simulink model "sys_model"  (R2015a)
settings: configuration reference "config_cosim" (kept outside this file)
InitFcn:
  | h  = findall(0, 'tag','Display');
  | close(h)
  | load TestVel
StartFcn:
  | Display
StopFcn:
  | h  = findall(0, 'tag','Display');
  | %close(h)
undefined symbols (not defined in the file): Vmsl, Vtgt
(part 1 of 2)
settings Model: CovModelRefEnable=off  Creator=The MathWorks, Inc.  LastModifiedBy=ericli
settings ConfigSetRef: SourceLocation=Base Workspace

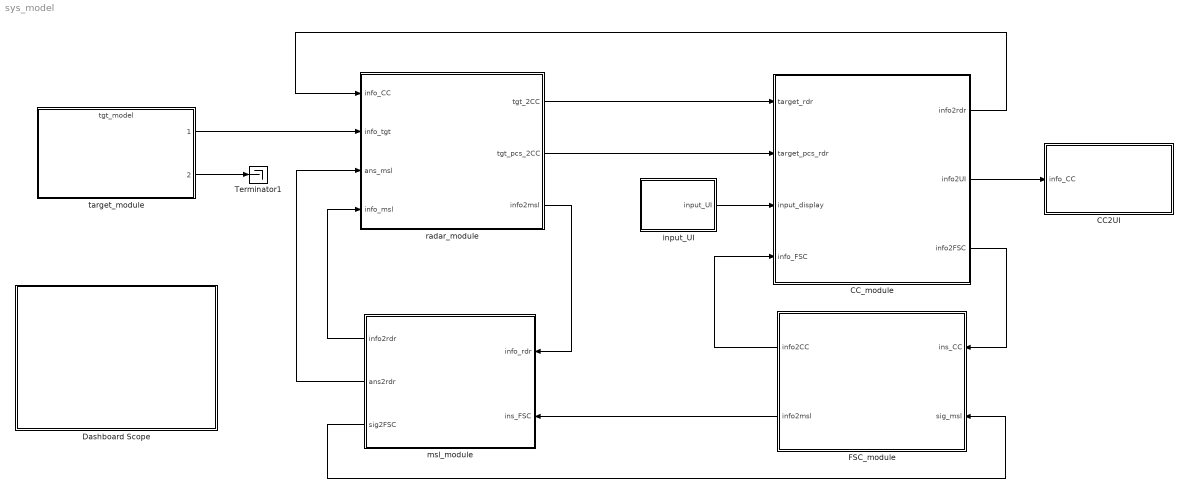
== system sys_model ==
  CC2UI : Subsystem
  CC_module : Subsystem
  Dashboard Scope : Subsystem  DialogController=hmiCreateDDGDialog  IsWebBlock=on  mask(MathWorksWebBlock){webBlockId=861919ea-88f4-4d9a-9fd6-bc31e51d36de, webBlockType=sdiscope, ShowInitialText=on, HMISrcModelName=sys_model}
      mask prompts: webBlockId "WebBlock Id"; webBlockType "WebBlock Type"; HMISrcModelName "Source Model"
      mask Help: helpview([docroot '/mapfiles/simulink.map'], 'hmi_scope')
      mask Display:
      | if strcmp(get_param(bdroot(gcb),'BlockDiagramType'), 'library')
      |     image([(matlabroot) '/toolbox/simulink/hmi/icons/DashboardScope.png']);
      | end
  FSC_module : Subsystem
  Terminator1 : Terminator
  input_UI : Subsystem
  msl_module : Subsystem
  radar_module : Subsystem
  target_module : ModelReference  ModelNameDialog=tgt_model.slx  SimulationMode=Normal  ModelReferenceVersion=1.185  CopyOfModelName=tgt_model.slx  DefaultDataLogging=on
  wires:
  target_module/1 -> radar_module/2(info_tgt)
  FSC_module/2(info2msl) -> msl_module/2(ins_FSC)
  CC_module/2(info2UI) -> CC2UI/1(info_CC)
  radar_module/3(info2msl) -> msl_module/1(info_rdr)
  msl_module/1(info2rdr) -> radar_module/4(info_msl)
  FSC_module/1(info2CC) -> CC_module/4(info_FSC)
  CC_module/1(info2rdr) -> radar_module/1(info_CC)
  target_module/2 -> Terminator1/1
  input_UI/1(input_UI) -> CC_module/3(input_display)
  msl_module/2(ans2rdr) -> radar_module/3(ans_msl)
  msl_module/3(sig2FSC) -> FSC_module/2(sig_msl)
  CC_module/3(info2FSC) -> FSC_module/1(ins_CC)
  radar_module/1(tgt_2CC) -> CC_module/1(target_rdr)
  radar_module/2(tgt_pcs_2CC) -> CC_module/2(target_pcs_rdr)

== system sys_model/CC2UI ==
  info_CC : Inport
  Bus Selector : BusSelector  OutputSignals=TargetData,AsnData,StateData,Avl_info,MslMotion
  Model : ModelReference  ModelNameDialog=SetData.slx  SimulationMode=Normal  ModelReferenceVersion=1.204  CopyOfModelName=SetData.slx  DefaultDataLogging=on
  wires:
  info_CC/1 -> Bus Selector/1
  Bus Selector/1 -> Model/1  "<TargetData>"
  Bus Selector/2 -> Model/2  "<AsnData>"
  Bus Selector/3 -> Model/3  "<StateData>"
  Bus Selector/4 -> Model/4  "<Avl_info>"
  Bus Selector/5 -> Model/5  "<MslMotion>"

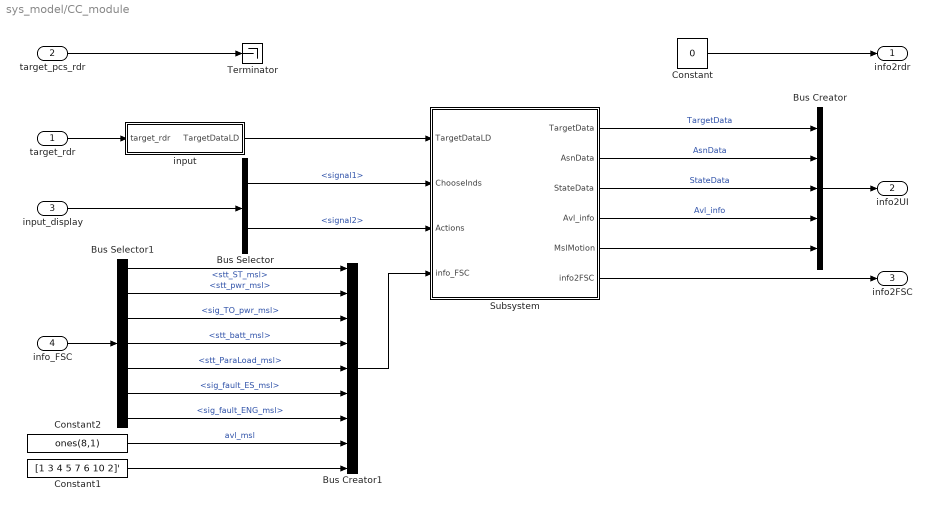
== system sys_model/CC_module ==
  target_rdr : Inport  OutDataTypeStr=Bus: BusObject_tgt_rdr2CC
  target_pcs_rdr : Inport  Port=2
  input_display : Inport  Port=3
  info_FSC : Inport  Port=4  OutDataTypeStr=Bus: BusObject_info_FSC2CC
  Bus Creator : BusCreator  Inputs=5
  Bus Creator1 : BusCreator  Inputs=9  OutDataTypeStr=Bus: BusObject_info_FSC2CC
  Bus Selector : BusSelector  OutputSignals=signal1,signal2
  Bus Selector1 : BusSelector  OutputSignals=stt_ST_msl,stt_pwr_msl,sig_TO_pwr_msl,stt_batt_msl,stt_ParaLoad_msl,sig_fault_ES_msl,sig_fault_ENG_msl
  Constant : Constant  Value=0  OutDataTypeStr=Bus:BusObject_info_CC2rdr  LockScale=on
  Constant1 : Constant  Value=[1 3 4 5 7 6 10 2]'  OutDataTypeStr=double
  Constant2 : Constant  Value=ones(8,1)  OutDataTypeStr=boolean
  Subsystem : Subsystem
  Terminator : Terminator
  input : Subsystem
  info2rdr : Outport  OutDataTypeStr=Bus: BusObject_info_CC2rdr
  info2UI : Outport  Port=2
  info2FSC : Outport  Port=3  OutDataTypeStr=Bus: BusObject_info_CC2FSC
  wires:
  Bus Creator/1 -> info2UI/1
  input_display/1 -> Bus Selector/1
  Bus Selector/2 -> Subsystem/3(Actions)  "<signal2>"
  Subsystem/6(info2FSC) -> info2FSC/1
  Constant/1 -> info2rdr/1
  Subsystem/4(Avl_info) -> Bus Creator/4  "Avl_info"
  Subsystem/3(StateData) -> Bus Creator/3  "StateData"
  Subsystem/1(TargetData) -> Bus Creator/1  "TargetData"
  input/1(TargetDataLD) -> Subsystem/1(TargetDataLD)
  target_pcs_rdr/1 -> Terminator/1
  Subsystem/2(AsnData) -> Bus Creator/2  "AsnData"
  info_FSC/1 -> Bus Selector1/1
  Bus Selector1/1 -> Bus Creator1/1  "<stt_ST_msl>"
  Bus Selector1/3 -> Bus Creator1/3  "<sig_TO_pwr_msl>"
  Bus Selector1/4 -> Bus Creator1/4  "<stt_batt_msl>"
  Bus Selector1/5 -> Bus Creator1/5  "<stt_ParaLoad_msl>"
  Bus Selector1/6 -> Bus Creator1/6  "<sig_fault_ES_msl>"
  Bus Selector1/7 -> Bus Creator1/7  "<sig_fault_ENG_msl>"
  Constant2/1 -> Bus Creator1/8  "avl_msl"
  Constant1/1 -> Bus Creator1/9
  Bus Creator1/1 -> Subsystem/4(info_FSC)
  target_rdr/1 -> input/1(target_rdr)
  Bus Selector/1 -> Subsystem/2(ChooseInds)  "<signal1>"
  Subsystem/5(MslMotion) -> Bus Creator/5
  Bus Selector1/2 -> Bus Creator1/2  "<stt_pwr_msl>"

== system sys_model/Dashboard Scope ==

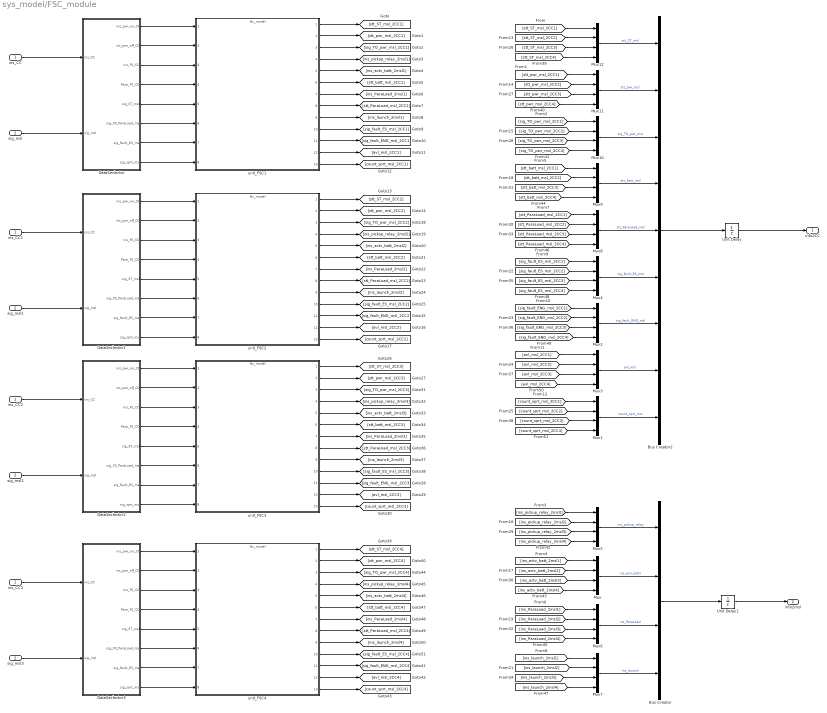
== system sys_model/FSC_module ==
  ins_CC : Inport
  sig_msl : Inport  Port=2
  Bus Creator : BusCreator  OutDataTypeStr=Bus: BusObject_info_FSC2msl  NonVirtualBus=on
      settings: InheritFromInputs=off
  Bus Creator2 : BusCreator  Inputs=9  OutDataTypeStr=Bus: BusObject_info_FSC2CC  NonVirtualBus=on
      settings: InheritFromInputs=off
  DataSeclector : Subsystem
  DataSeclector1 : Subsystem
  DataSeclector2 : Subsystem
  DataSeclector3 : Subsystem
  Mux{,1..12} (13 alike) : Mux
  Unit Delay : UnitDelay  SampleTime=-1
  Unit Delay1 : UnitDelay  SampleTime=-1
  ins_CC1 : InportShadow
  ins_CC2 : InportShadow
  ins_CC3 : InportShadow
  sig_msl1 : InportShadow  Port=2
  sig_msl2 : InportShadow  Port=2
  sig_msl3 : InportShadow  Port=2
  unit_FSC{1..4} (4 alike) : ModelReference  ModelNameDialog=fsc_model.slx  SimulationMode=Normal  ModelReferenceVersion=1.143  CopyOfModelName=fsc_model.slx  DefaultDataLogging=on
  info2CC : Outport  OutDataTypeStr=Bus: BusObject_info_FSC2CC
  info2msl : Outport  Port=2  OutDataTypeStr=Bus: BusObject_info_FSC2msl
  wires:
  unit_FSC1/1 -> [stt_ST_msl_2CC1]
  unit_FSC1/2 -> [stt_pwr_msl_2CC1]
  unit_FSC1/3 -> [sig_TO_pwr_msl_2CC1]
  unit_FSC1/4 -> [ins_pickup_relay_2msl1]
  unit_FSC1/5 -> [ins_actv_batt_2msl1]
  unit_FSC1/6 -> [stt_batt_msl_2CC1]
  unit_FSC1/7 -> [ins_ParaLoad_2msl1]
  unit_FSC1/8 -> [stt_ParaLoad_msl_2CC1]
  unit_FSC1/9 -> [ins_launch_2msl1]
  unit_FSC1/10 -> [sig_fault_ES_msl_2CC1]
  unit_FSC1/11 -> [sig_fault_ENG_msl_2CC1]
  unit_FSC1/12 -> [avl_msl_2CC1]
  unit_FSC1/13 -> [count_sprt_msl_2CC1]
  unit_FSC2/13 -> [count_sprt_msl_2CC2]
  unit_FSC2/6 -> [stt_batt_msl_2CC2]
  unit_FSC2/10 -> [sig_fault_ES_msl_2CC2]
  unit_FSC2/3 -> [sig_TO_pwr_msl_2CC2]
  unit_FSC2/7 -> [ins_ParaLoad_2msl2]
  unit_FSC2/11 -> [sig_fault_ENG_msl_2CC2]
  unit_FSC2/4 -> [ins_pickup_relay_2msl2]
  unit_FSC2/8 -> [stt_ParaLoad_msl_2CC2]
  unit_FSC2/1 -> [stt_ST_msl_2CC2]
  unit_FSC2/2 -> [stt_pwr_msl_2CC2]
  unit_FSC2/9 -> [ins_launch_2msl2]
  unit_FSC2/12 -> [avl_msl_2CC2]
  unit_FSC2/5 -> [ins_actv_batt_2msl2]
  unit_FSC3/11 -> [sig_fault_ENG_msl_2CC3]
  unit_FSC3/7 -> [ins_ParaLoad_2msl3]
  unit_FSC3/4 -> [ins_pickup_relay_2msl3]
  unit_FSC3/10 -> [sig_fault_ES_msl_2CC3]
  unit_FSC3/5 -> [ins_actv_batt_2msl3]
  unit_FSC3/6 -> [stt_batt_msl_2CC3]
  unit_FSC3/3 -> [sig_TO_pwr_msl_2CC3]
  unit_FSC3/1 -> [stt_ST_msl_2CC3]
  unit_FSC3/13 -> [count_sprt_msl_2CC3]
  unit_FSC3/12 -> [avl_msl_2CC3]
  unit_FSC3/2 -> [stt_pwr_msl_2CC3]
  unit_FSC3/9 -> [ins_launch_2msl3]
  unit_FSC3/8 -> [stt_ParaLoad_msl_2CC3]
  unit_FSC4/11 -> [sig_fault_ENG_msl_2CC4]
  unit_FSC4/12 -> [avl_msl_2CC4]
  unit_FSC4/10 -> [sig_fault_ES_msl_2CC4]
  unit_FSC4/9 -> [ins_launch_2msl4]
  unit_FSC4/8 -> [stt_ParaLoad_msl_2CC4]
  unit_FSC4/7 -> [ins_ParaLoad_2msl4]
  unit_FSC4/6 -> [stt_batt_msl_2CC4]
  unit_FSC4/5 -> [ins_actv_batt_2msl4]
  unit_FSC4/4 -> [ins_pickup_relay_2msl4]
  unit_FSC4/3 -> [sig_TO_pwr_msl_2CC4]
  unit_FSC4/1 -> [stt_ST_msl_2CC4]
  unit_FSC4/2 -> [stt_pwr_msl_2CC4]
  unit_FSC4/13 -> [count_sprt_msl_2CC4]
  [stt_ST_msl_2CC1] -> Mux12/1
  [stt_ST_msl_2CC2] -> Mux12/2
  [stt_ST_msl_2CC3] -> Mux12/3
  [stt_ST_msl_2CC4] -> Mux12/4
  [stt_pwr_msl_2CC1] -> Mux11/1
  [stt_pwr_msl_2CC2] -> Mux11/2
  [stt_pwr_msl_2CC3] -> Mux11/3
  [stt_pwr_msl_2CC4] -> Mux11/4
  [sig_TO_pwr_msl_2CC1] -> Mux10/1
  [sig_TO_pwr_msl_2CC2] -> Mux10/2
  [sig_TO_pwr_msl_2CC3] -> Mux10/3
  [sig_TO_pwr_msl_2CC4] -> Mux10/4
  [ins_pickup_relay_2msl1] -> Mux5/1
  [ins_pickup_relay_2msl2] -> Mux5/2
  [ins_pickup_relay_2msl3] -> Mux5/3
  [ins_pickup_relay_2msl4] -> Mux5/4
  [ins_actv_batt_2msl1] -> Mux/1
  [ins_actv_batt_2msl2] -> Mux/2
  [ins_actv_batt_2msl3] -> Mux/3
  [ins_actv_batt_2msl4] -> Mux/4
  [stt_batt_msl_2CC1] -> Mux9/1
  [stt_batt_msl_2CC2] -> Mux9/2
  [stt_batt_msl_2CC3] -> Mux9/3
  [stt_batt_msl_2CC4] -> Mux9/4
  [ins_ParaLoad_2msl1] -> Mux6/1
  [ins_ParaLoad_2msl2] -> Mux6/2
  [ins_ParaLoad_2msl3] -> Mux6/3
  [ins_ParaLoad_2msl4] -> Mux6/4
  [stt_ParaLoad_msl_2CC1] -> Mux8/1
  [stt_ParaLoad_msl_2CC2] -> Mux8/2
  [stt_ParaLoad_msl_2CC3] -> Mux8/3
  [stt_ParaLoad_msl_2CC4] -> Mux8/4
  [ins_launch_2msl1] -> Mux7/1
  [ins_launch_2msl2] -> Mux7/2
  [ins_launch_2msl3] -> Mux7/3
  [ins_launch_2msl4] -> Mux7/4
  [sig_fault_ES_msl_2CC1] -> Mux4/1
  [sig_fault_ES_msl_2CC2] -> Mux4/2
  [sig_fault_ES_msl_2CC3] -> Mux4/3
  [sig_fault_ES_msl_2CC4] -> Mux4/4
  [sig_fault_ENG_msl_2CC1] -> Mux2/1
  [sig_fault_ENG_msl_2CC2] -> Mux2/2
  [sig_fault_ENG_msl_2CC3] -> Mux2/3
  [sig_fault_ENG_msl_2CC4] -> Mux2/4
  [avl_msl_2CC1] -> Mux3/1
  [avl_msl_2CC2] -> Mux3/2
  [avl_msl_2CC3] -> Mux3/3
  [avl_msl_2CC4] -> Mux3/4
  [count_sprt_msl_2CC1] -> Mux1/1
  [count_sprt_msl_2CC2] -> Mux1/2
  [count_sprt_msl_2CC3] -> Mux1/3
  [count_sprt_msl_2CC4] -> Mux1/4
  Mux6/1 -> Bus Creator/3  "ins_ParaLoad"
  Mux/1 -> Bus Creator/2  "ins_actv_batt"
  Mux7/1 -> Bus Creator/4  "ins_launch"
  Mux5/1 -> Bus Creator/1  "ins_pickup_relay"
  Bus Creator/1 -> Unit Delay1/1
  Mux10/1 -> Bus Creator2/3  "sig_TO_pwr_msl"
  Mux9/1 -> Bus Creator2/4  "stt_batt_msl"
  Mux11/1 -> Bus Creator2/2  "stt_pwr_msl"
  Mux8/1 -> Bus Creator2/5  "stt_ParaLoad_msl"
  Mux4/1 -> Bus Creator2/6  "sig_fault_ES_msl"
  Mux12/1 -> Bus Creator2/1  "stt_ST_msl"
  Mux2/1 -> Bus Creator2/7  "sig_fault_ENG_msl"
  Mux3/1 -> Bus Creator2/8  "avl_msl"
  Mux1/1 -> Bus Creator2/9  "count_sprt_msl"
  Bus Creator2/1 -> Unit Delay/1
  ins_CC/1 -> DataSeclector/1(ins_CC)
  sig_msl/1 -> DataSeclector/2(sig_msl)
  DataSeclector/3(ins_FS_CC) -> unit_FSC1/3
  DataSeclector/2(ins_pwr_off_CC) -> unit_FSC1/2
  DataSeclector/4(Para_FS_CC) -> unit_FSC1/4
  DataSeclector/5(sig_ST_msl) -> unit_FSC1/5
  DataSeclector/1(ins_pwr_on_CC) -> unit_FSC1/1
  DataSeclector/6(sig_CK_ParaLoad_msl) -> unit_FSC1/6
  DataSeclector/7(sig_fault_ES_msl) -> unit_FSC1/7
  DataSeclector/8(sig_sprt_msl) -> unit_FSC1/8
  DataSeclector3/6(sig_CK_ParaLoad_msl) -> unit_FSC4/6
  DataSeclector3/2(ins_pwr_off_CC) -> unit_FSC4/2
  DataSeclector3/5(sig_ST_msl) -> unit_FSC4/5
  DataSeclector3/8(sig_sprt_msl) -> unit_FSC4/8
  DataSeclector3/4(Para_FS_CC) -> unit_FSC4/4
  DataSeclector3/3(ins_FS_CC) -> unit_FSC4/3
  DataSeclector3/1(ins_pwr_on_CC) -> unit_FSC4/1
  DataSeclector3/7(sig_fault_ES_msl) -> unit_FSC4/7
  DataSeclector2/4(Para_FS_CC) -> unit_FSC3/4
  DataSeclector2/2(ins_pwr_off_CC) -> unit_FSC3/2
  DataSeclector2/1(ins_pwr_on_CC) -> unit_FSC3/1
  DataSeclector2/5(sig_ST_msl) -> unit_FSC3/5
  DataSeclector2/3(ins_FS_CC) -> unit_FSC3/3
  DataSeclector2/7(sig_fault_ES_msl) -> unit_FSC3/7
  DataSeclector2/8(sig_sprt_msl) -> unit_FSC3/8
  DataSeclector2/6(sig_CK_ParaLoad_msl) -> unit_FSC3/6
  DataSeclector1/8(sig_sprt_msl) -> unit_FSC2/8
  DataSeclector1/1(ins_pwr_on_CC) -> unit_FSC2/1
  DataSeclector1/6(sig_CK_ParaLoad_msl) -> unit_FSC2/6
  DataSeclector1/4(Para_FS_CC) -> unit_FSC2/4
  DataSeclector1/3(ins_FS_CC) -> unit_FSC2/3
  DataSeclector1/5(sig_ST_msl) -> unit_FSC2/5
  DataSeclector1/7(sig_fault_ES_msl) -> unit_FSC2/7
  DataSeclector1/2(ins_pwr_off_CC) -> unit_FSC2/2
  sig_msl1/1 -> DataSeclector1/2(sig_msl)
  ins_CC1/1 -> DataSeclector1/1(ins_CC)
  ins_CC2/1 -> DataSeclector2/1(ins_CC)
  sig_msl2/1 -> DataSeclector2/2(sig_msl)
  sig_msl3/1 -> DataSeclector3/2(sig_msl)
  ins_CC3/1 -> DataSeclector3/1(ins_CC)
  Unit Delay/1 -> info2CC/1
  Unit Delay1/1 -> info2msl/1

== system sys_model/input_UI ==
  " get_input_UI" : ModelReference  ModelNameDialog=input_display.slx  SimulationMode=Normal  ModelReferenceVersion=1.222  CopyOfModelName=input_display.slx  DefaultDataLogging=on
  Bus Creator : BusCreator  Inputs=2
  input_UI : Outport
  wires:
  Bus Creator/1 -> input_UI/1
  " get_input_UI"/1 -> Bus Creator/1
  " get_input_UI"/2 -> Bus Creator/2

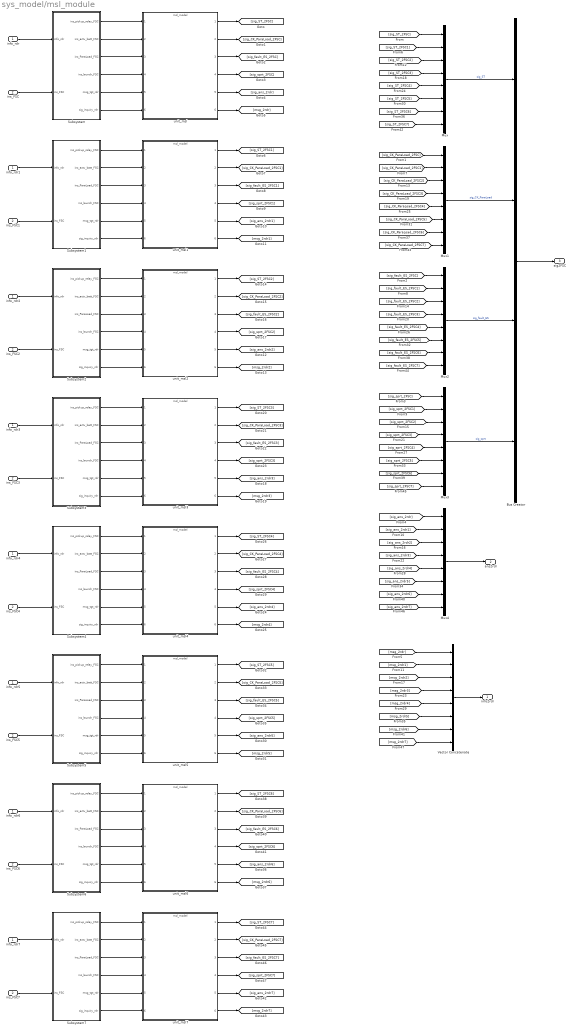
== system sys_model/msl_module ==
  info_rdr : Inport
  ins_FSC : Inport  Port=2
  Bus Creator : BusCreator
  Mux{,1..4} (5 alike) : Mux  Inputs=8
  Subsystem : Subsystem
  Subsystem1 : Subsystem
  Subsystem2 : Subsystem
  Subsystem3 : Subsystem
  Subsystem4 : Subsystem
  Subsystem5 : Subsystem
  Subsystem6 : Subsystem
  Subsystem7 : Subsystem
  Vector Concatenate : Concatenate  NumInputs=8
  info_rdr{1..7} (7 alike) : InportShadow
  ins_FSC{1..7} (7 alike) : InportShadow  Port=2
  unit_msl{,1..7} (8 alike) : ModelReference  ModelNameDialog=msl_model.slx  SimulationMode=Normal  ModelReferenceVersion=1.166  CopyOfModelName=msl_model.slx  DefaultDataLogging=on
  info2rdr : Outport  OutDataTypeStr=Bus: BusObject_msg_msl2rdr
  ans2rdr : Outport  Port=2
  sig2FSC : Outport  Port=3  OutDataTypeStr=Bus: BusObject_info_msl2FSC
  wires:
  ins_FSC/1 -> Subsystem/2(ins_FSC)
  info_rdr/1 -> Subsystem/1(info_rdr)
  Subsystem/1(ins_pickup_relay_FSC) -> unit_msl/1
  Subsystem/2(ins_actv_batt_FSC) -> unit_msl/2
  Subsystem/3(ins_ParaLoad_FSC) -> unit_msl/3
  Subsystem/4(ins_launch_FSC) -> unit_msl/4
  Subsystem/5(msg_tgt_rdr) -> unit_msl/5
  Subsystem/6(sig_inquiry_rdr) -> unit_msl/6
  ins_FSC1/1 -> Subsystem1/2(ins_FSC)
  info_rdr1/1 -> Subsystem1/1(info_rdr)
  Subsystem1/1(ins_pickup_relay_FSC) -> unit_msl1/1
  Subsystem1/2(ins_actv_batt_FSC) -> unit_msl1/2
  Subsystem1/3(ins_ParaLoad_FSC) -> unit_msl1/3
  Subsystem1/4(ins_launch_FSC) -> unit_msl1/4
  Subsystem1/5(msg_tgt_rdr) -> unit_msl1/5
  Subsystem1/6(sig_inquiry_rdr) -> unit_msl1/6
  ins_FSC2/1 -> Subsystem2/2(ins_FSC)
  info_rdr2/1 -> Subsystem2/1(info_rdr)
  Subsystem2/1(ins_pickup_relay_FSC) -> unit_msl2/1
  Subsystem2/2(ins_actv_batt_FSC) -> unit_msl2/2
  Subsystem2/3(ins_ParaLoad_FSC) -> unit_msl2/3
  Subsystem2/4(ins_launch_FSC) -> unit_msl2/4
  Subsystem2/5(msg_tgt_rdr) -> unit_msl2/5
  Subsystem2/6(sig_inquiry_rdr) -> unit_msl2/6
  ins_FSC3/1 -> Subsystem3/2(ins_FSC)
  info_rdr3/1 -> Subsystem3/1(info_rdr)
  Subsystem3/1(ins_pickup_relay_FSC) -> unit_msl3/1
  Subsystem3/2(ins_actv_batt_FSC) -> unit_msl3/2
  Subsystem3/3(ins_ParaLoad_FSC) -> unit_msl3/3
  Subsystem3/4(ins_launch_FSC) -> unit_msl3/4
  Subsystem3/5(msg_tgt_rdr) -> unit_msl3/5
  Subsystem3/6(sig_inquiry_rdr) -> unit_msl3/6
  ins_FSC4/1 -> Subsystem4/2(ins_FSC)
  info_rdr4/1 -> Subsystem4/1(info_rdr)
  Subsystem4/1(ins_pickup_relay_FSC) -> unit_msl4/1
  Subsystem4/2(ins_actv_batt_FSC) -> unit_msl4/2
  Subsystem4/3(ins_ParaLoad_FSC) -> unit_msl4/3
  Subsystem4/4(ins_launch_FSC) -> unit_msl4/4
  Subsystem4/5(msg_tgt_rdr) -> unit_msl4/5
  Subsystem4/6(sig_inquiry_rdr) -> unit_msl4/6
  ins_FSC5/1 -> Subsystem5/2(ins_FSC)
  info_rdr5/1 -> Subsystem5/1(info_rdr)
  Subsystem5/1(ins_pickup_relay_FSC) -> unit_msl5/1
  Subsystem5/2(ins_actv_batt_FSC) -> unit_msl5/2
  Subsystem5/3(ins_ParaLoad_FSC) -> unit_msl5/3
  Subsystem5/4(ins_launch_FSC) -> unit_msl5/4
  Subsystem5/5(msg_tgt_rdr) -> unit_msl5/5
  Subsystem5/6(sig_inquiry_rdr) -> unit_msl5/6
  ins_FSC6/1 -> Subsystem6/2(ins_FSC)
  info_rdr6/1 -> Subsystem6/1(info_rdr)
  Subsystem6/1(ins_pickup_relay_FSC) -> unit_msl6/1
  Subsystem6/2(ins_actv_batt_FSC) -> unit_msl6/2
  Subsystem6/3(ins_ParaLoad_FSC) -> unit_msl6/3
  Subsystem6/4(ins_launch_FSC) -> unit_msl6/4
  Subsystem6/5(msg_tgt_rdr) -> unit_msl6/5
  Subsystem6/6(sig_inquiry_rdr) -> unit_msl6/6
  ins_FSC7/1 -> Subsystem7/2(ins_FSC)
  info_rdr7/1 -> Subsystem7/1(info_rdr)
  Subsystem7/1(ins_pickup_relay_FSC) -> unit_msl7/1
  Subsystem7/2(ins_actv_batt_FSC) -> unit_msl7/2
  Subsystem7/3(ins_ParaLoad_FSC) -> unit_msl7/3
  Subsystem7/4(ins_launch_FSC) -> unit_msl7/4
  Subsystem7/5(msg_tgt_rdr) -> unit_msl7/5
  Subsystem7/6(sig_inquiry_rdr) -> unit_msl7/6
  unit_msl/1 -> [sig_ST_2FSC]
  unit_msl/2 -> [sig_CK_ParaLoad_2FSC]
  unit_msl/3 -> [sig_fault_ES_2FSC]
  unit_msl/4 -> [sig_sprt_2FSC]
  unit_msl/5 -> [sig_ans_2rdr]
  unit_msl/6 -> [msg_2rdr]
  unit_msl1/1 -> [sig_ST_2FSC1]
  unit_msl1/2 -> [sig_CK_ParaLoad_2FSC1]
  unit_msl1/3 -> [sig_fault_ES_2FSC1]
  unit_msl1/4 -> [sig_sprt_2FSC1]
  unit_msl1/5 -> [sig_ans_2rdr1]
  unit_msl1/6 -> [msg_2rdr1]
  unit_msl2/1 -> [sig_ST_2FSC2]
  unit_msl2/2 -> [sig_CK_ParaLoad_2FSC2]
  unit_msl2/3 -> [sig_fault_ES_2FSC2]
  unit_msl2/4 -> [sig_sprt_2FSC2]
  unit_msl2/5 -> [sig_ans_2rdr2]
  unit_msl2/6 -> [msg_2rdr2]
  unit_msl3/1 -> [sig_ST_2FSC3]
  unit_msl3/2 -> [sig_CK_ParaLoad_2FSC3]
  unit_msl3/3 -> [sig_fault_ES_2FSC3]
  unit_msl3/4 -> [sig_sprt_2FSC3]
  unit_msl3/5 -> [sig_ans_2rdr3]
  unit_msl3/6 -> [msg_2rdr3]
  unit_msl4/1 -> [sig_ST_2FSC4]
  unit_msl4/2 -> [sig_CK_ParaLoad_2FSC4]
  unit_msl4/3 -> [sig_fault_ES_2FSC4]
  unit_msl4/4 -> [sig_sprt_2FSC4]
  unit_msl4/5 -> [sig_ans_2rdr4]
  unit_msl4/6 -> [msg_2rdr4]
  unit_msl5/1 -> [sig_ST_2FSC5]
  unit_msl5/2 -> [sig_CK_ParaLoad_2FSC5]
  unit_msl5/3 -> [sig_fault_ES_2FSC5]
  unit_msl5/4 -> [sig_sprt_2FSC5]
  unit_msl5/5 -> [sig_ans_2rdr5]
  unit_msl5/6 -> [msg_2rdr5]
  unit_msl6/1 -> [sig_ST_2FSC6]
  unit_msl6/2 -> [sig_CK_ParaLoad_2FSC6]
  unit_msl6/3 -> [sig_fault_ES_2FSC6]
  unit_msl6/4 -> [sig_sprt_2FSC6]
  unit_msl6/5 -> [sig_ans_2rdr6]
  unit_msl6/6 -> [msg_2rdr6]
  unit_msl7/1 -> [sig_ST_2FSC7]
  unit_msl7/2 -> [sig_CK_ParaLoad_2FSC7]
  unit_msl7/3 -> [sig_fault_ES_2FSC7]
  unit_msl7/4 -> [sig_sprt_2FSC7]
  unit_msl7/5 -> [sig_ans_2rdr7]
  unit_msl7/6 -> [msg_2rdr7]
  [sig_ST_2FSC5] -> Mux/6
  [sig_ST_2FSC3] -> Mux/4
  [sig_ST_2FSC6] -> Mux/7
  [sig_ST_2FSC2] -> Mux/3
  [sig_ST_2FSC4] -> Mux/5
  [sig_ST_2FSC7] -> Mux/8
  [sig_ST_2FSC] -> Mux/1
  [sig_ST_2FSC1] -> Mux/2
  [sig_CK_ParaLoad_2FSC2] -> Mux1/3
  [sig_CK_ParaLoad_2FSC4] -> Mux1/5
  [sig_CK_ParaLoad_2FSC3] -> Mux1/4
  [sig_CK_ParaLoad_2FSC7] -> Mux1/8
  [sig_CK_ParaLoad_2FSC5] -> Mux1/6
  [sig_CK_ParaLoad_2FSC6] -> Mux1/7
  [sig_CK_ParaLoad_2FSC] -> Mux1/1
  [sig_CK_ParaLoad_2FSC1] -> Mux1/2
  [sig_fault_ES_2FSC5] -> Mux2/6
  [sig_fault_ES_2FSC1] -> Mux2/2
  [sig_fault_ES_2FSC4] -> Mux2/5
  [sig_fault_ES_2FSC6] -> Mux2/7
  [sig_fault_ES_2FSC2] -> Mux2/3
  [sig_fault_ES_2FSC3] -> Mux2/4
  [sig_fault_ES_2FSC7] -> Mux2/8
  [sig_fault_ES_2FSC] -> Mux2/1
  [sig_sprt_2FSC2] -> Mux3/3
  [sig_sprt_2FSC4] -> Mux3/5
  [sig_sprt_2FSC7] -> Mux3/8
  [sig_sprt_2FSC1] -> Mux3/2
  [sig_sprt_2FSC5] -> Mux3/6
  [sig_sprt_2FSC3] -> Mux3/4
  [sig_sprt_2FSC] -> Mux3/1
  [sig_sprt_2FSC6] -> Mux3/7
  [sig_ans_2rdr4] -> Mux4/5
  [sig_ans_2rdr5] -> Mux4/6
  [sig_ans_2rdr] -> Mux4/1
  [sig_ans_2rdr7] -> Mux4/8
  [sig_ans_2rdr6] -> Mux4/7
  [sig_ans_2rdr2] -> Mux4/3
  [sig_ans_2rdr3] -> Mux4/4
  [sig_ans_2rdr1] -> Mux4/2
  [msg_2rdr] -> Vector Concatenate/1
  [msg_2rdr2] -> Vector Concatenate/3
  [msg_2rdr1] -> Vector Concatenate/2
  [msg_2rdr4] -> Vector Concatenate/5
  [msg_2rdr3] -> Vector Concatenate/4
  [msg_2rdr6] -> Vector Concatenate/7
  [msg_2rdr7] -> Vector Concatenate/8
  [msg_2rdr5] -> Vector Concatenate/6
  Mux/1 -> Bus Creator/1  "sig_ST"
  Mux1/1 -> Bus Creator/2  "sig_CK_ParaLoad"
  Mux2/1 -> Bus Creator/3  "sig_fault_ES"
  Mux3/1 -> Bus Creator/4  "sig_sprt"
  Bus Creator/1 -> sig2FSC/1
  Mux4/1 -> ans2rdr/1
  Vector Concatenate/1 -> info2rdr/1

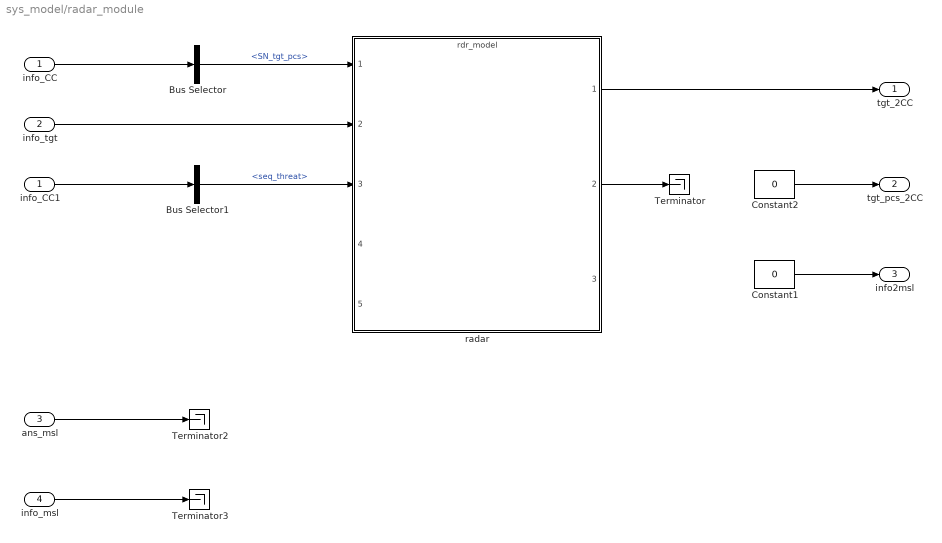
== system sys_model/radar_module ==
  info_CC : Inport
  info_tgt : Inport  Port=2  PortDimensions=100  BusOutputAsStruct=on
  ans_msl : Inport  Port=3
  info_msl : Inport  Port=4
  Bus Selector : BusSelector  OutputSignals=SN_tgt_pcs
  Bus Selector1 : BusSelector  OutputSignals=seq_threat
  Constant1 : Constant  Value=0  OutDataTypeStr=Bus: BusObject_info_rdr2msl
  Constant2 : Constant  Value=0  OutDataTypeStr=Bus: BusObject_msg_pcs_rdr2CC
  Terminator : Terminator
  Terminator2 : Terminator
  Terminator3 : Terminator
  info_CC1 : InportShadow
  radar : ModelReference  ModelNameDialog=rdr_model.slx  SimulationMode=Normal  ModelReferenceVersion=1.187  CopyOfModelName=rdr_model.slx  DefaultDataLogging=on
  tgt_2CC : Outport  OutDataTypeStr=Bus: BusObject_tgt_rdr2CC
  tgt_pcs_2CC : Outport  Port=2  OutDataTypeStr=Bus: BusObject_msg_pcs_rdr2CC
  info2msl : Outport  Port=3  OutDataTypeStr=Bus: BusObject_info_rdr2msl
  wires:
  info_CC/1 -> Bus Selector/1
  Constant2/1 -> tgt_pcs_2CC/1
  Constant1/1 -> info2msl/1
  info_msl/1 -> Terminator3/1
  ans_msl/1 -> Terminator2/1
  info_tgt/1 -> radar/2
  Bus Selector/1 -> radar/1  "<SN_tgt_pcs>"
  radar/1 -> tgt_2CC/1
  radar/2 -> Terminator/1
  Bus Selector1/1 -> radar/3  "<seq_threat>"
  info_CC1/1 -> Bus Selector1/1

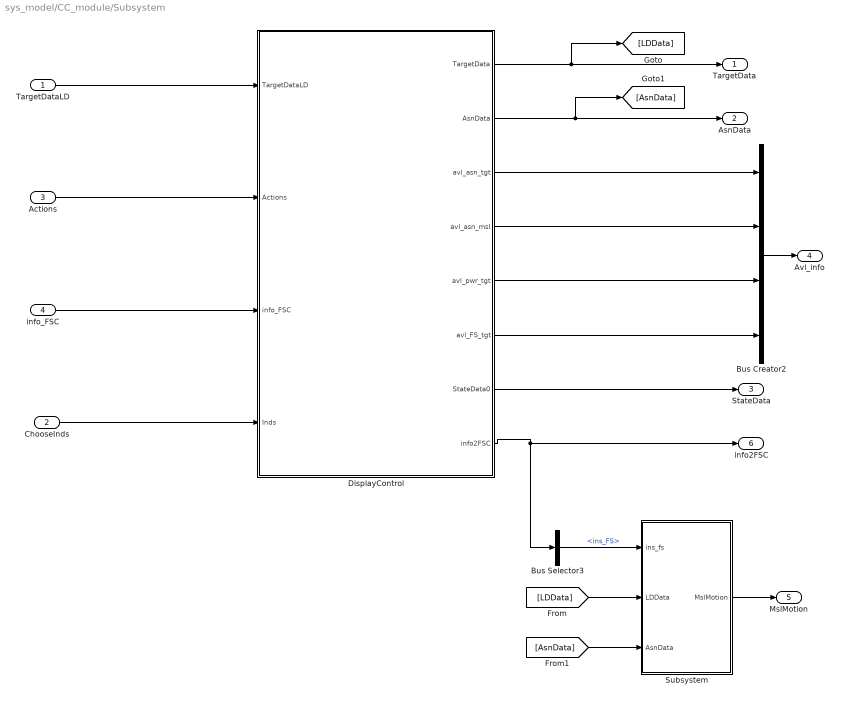
== system sys_model/CC_module/Subsystem ==
  TargetDataLD : Inport
  ChooseInds : Inport  Port=2  OutDataTypeStr=Bus:ChooseBusObject
  Actions : Inport  Port=3  OutDataTypeStr=Bus: ActionBusObject
  info_FSC : Inport  Port=4  OutDataTypeStr=Bus:BusObject_info_FSC2CC
  Bus Creator2 : BusCreator  OutDataTypeStr=Bus:AvlBusObject
  Bus Selector3 : BusSelector  OutputSignals=ins_FS
  DisplayControl : Stateflow chart  TreatAsAtomicUnit=on
  Subsystem : Subsystem
  TargetData : Outport
  AsnData : Outport  Port=2
  StateData : Outport  Port=3  OutDataTypeStr=Bus:StateBusObject
  Avl_info : Outport  Port=4  OutDataTypeStr=Bus:AvlBusObject
  MslMotion : Outport  Port=5  OutDataTypeStr=Bus: MslDataBusObject
  info2FSC : Outport  Port=6  OutDataTypeStr=Bus: BusObject_info_CC2FSC
  wires:
  DisplayControl/3(avl_asn_tgt) -> Bus Creator2/1
  DisplayControl/8(info2FSC) -> Bus Selector3/1, info2FSC/1
  DisplayControl/1(TargetData) -> [LDData], TargetData/1
  Bus Creator2/1 -> Avl_info/1
  TargetDataLD/1 -> DisplayControl/1(TargetDataLD)
  DisplayControl/5(avl_pwr_tgt) -> Bus Creator2/3
  DisplayControl/7(StateData0) -> StateData/1
  DisplayControl/4(avl_asn_msl) -> Bus Creator2/2
  DisplayControl/6(avl_FS_tgt) -> Bus Creator2/4
  Actions/1 -> DisplayControl/2(Actions)
  info_FSC/1 -> DisplayControl/3(info_FSC)
  DisplayControl/2(AsnData) -> [AsnData], AsnData/1
  [LDData] -> Subsystem/2(LDData)
  [AsnData] -> Subsystem/3(AsnData)
  Bus Selector3/1 -> Subsystem/1(ins_fs)  "<ins_FS>"
  Subsystem/1(MslMotion) -> MslMotion/1
  ChooseInds/1 -> DisplayControl/4(Inds)

== system sys_model/CC_module/input ==
  target_rdr : Inport  OutDataTypeStr=Bus: BusObject_tgt_rdr2CC
  Bus Creator1 : BusCreator  Inputs=3  OutDataTypeStr=Bus: TgtDataLDBusObject  NonVirtualBus=on
  Constant : Constant  Value=[1 3 4 5 7 6 10 2]'  OutDataTypeStr=double
  Constant1 : Constant  Value=[1:8]
  For Each Subsystem : Subsystem  TreatAsAtomicUnit=on
  Math Function : Math  Operator=transpose  SaturateOnIntegerOverflow=on
  Math Function1 : Math  Operator=transpose  SaturateOnIntegerOverflow=on
  Selector1 : Selector  InputPortWidth=48  IndexOptions=Index vector (port)  Indices=[1 3]
  TargetGeneration : Subsystem
  Terminator : Terminator
  Terminator1 : Terminator
  TargetDataLD : Outport  OutDataTypeStr=Bus: TgtDataLDBusObject
  wires:
  Constant/1 -> Bus Creator1/1  "Index"
  Bus Creator1/1 -> TargetDataLD/1
  target_rdr/1 -> Selector1/1
  Constant1/1 -> Selector1/2
  For Each Subsystem/2(vel) -> Math Function/1
  Selector1/1 -> For Each Subsystem/1(In1)
  For Each Subsystem/1(pos) -> Math Function1/1
  Math Function1/1 -> Terminator/1  "Pos"
  Math Function/1 -> Terminator1/1  "Vel"
  TargetGeneration/1(Pos) -> Bus Creator1/2
  TargetGeneration/2(Vel) -> Bus Creator1/3

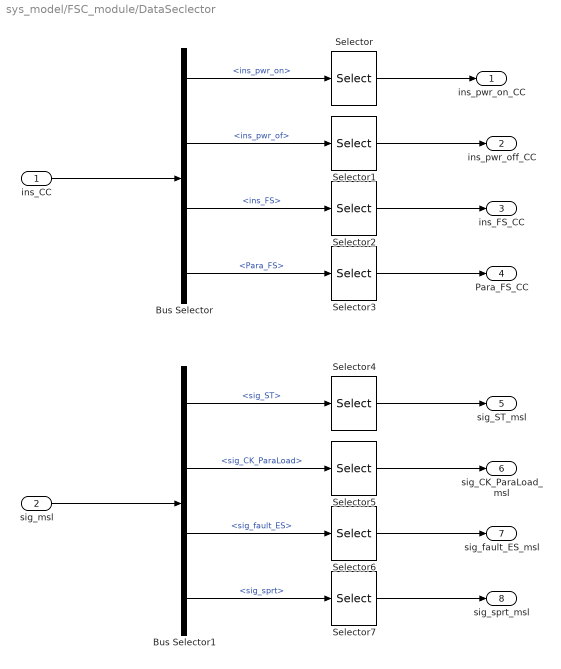
== system sys_model/FSC_module/DataSeclector ==
  ins_CC : Inport
  sig_msl : Inport  Port=2
  Bus Selector : BusSelector  OutputSignals=ins_pwr_on,ins_pwr_of,ins_FS,Para_FS
  Bus Selector1 : BusSelector  OutputSignals=sig_ST,sig_CK_ParaLoad,sig_fault_ES,sig_sprt
  Selector{,1..7} (8 alike) : Selector  InputPortWidth=8  Indices=[1 2]
  ins_pwr_on_CC : Outport
  ins_pwr_off_CC : Outport  Port=2
  ins_FS_CC : Outport  Port=3
  Para_FS_CC : Outport  Port=4
  sig_ST_msl : Outport  Port=5
  sig_CK_ParaLoad_msl : Outport  Port=6
  sig_fault_ES_msl : Outport  Port=7
  sig_sprt_msl : Outport  Port=8
  wires:
  ins_CC/1 -> Bus Selector/1
  sig_msl/1 -> Bus Selector1/1
  Bus Selector/1 -> Selector/1  "<ins_pwr_on>"
  Bus Selector/2 -> Selector1/1  "<ins_pwr_of>"
  Bus Selector/3 -> Selector2/1  "<ins_FS>"
  Bus Selector/4 -> Selector3/1  "<Para_FS>"
  Bus Selector1/1 -> Selector4/1  "<sig_ST>"
  Bus Selector1/2 -> Selector5/1  "<sig_CK_ParaLoad>"
  Bus Selector1/3 -> Selector6/1  "<sig_fault_ES>"
  Bus Selector1/4 -> Selector7/1  "<sig_sprt>"
  Selector/1 -> ins_pwr_on_CC/1
  Selector1/1 -> ins_pwr_off_CC/1
  Selector2/1 -> ins_FS_CC/1
  Selector3/1 -> Para_FS_CC/1
  Selector4/1 -> sig_ST_msl/1
  Selector5/1 -> sig_CK_ParaLoad_msl/1
  Selector6/1 -> sig_fault_ES_msl/1
  Selector7/1 -> sig_sprt_msl/1

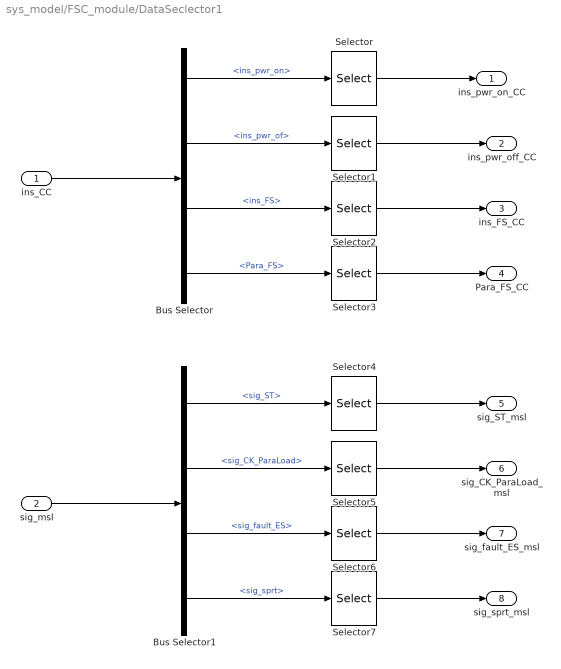
== system sys_model/FSC_module/DataSeclector1 ==
  ins_CC : Inport
  sig_msl : Inport  Port=2
  Bus Selector : BusSelector  OutputSignals=ins_pwr_on,ins_pwr_of,ins_FS,Para_FS
  Bus Selector1 : BusSelector  OutputSignals=sig_ST,sig_CK_ParaLoad,sig_fault_ES,sig_sprt
  Selector{,1..7} (8 alike) : Selector  InputPortWidth=8  Indices=[3 4]
  ins_pwr_on_CC : Outport
  ins_pwr_off_CC : Outport  Port=2
  ins_FS_CC : Outport  Port=3
  Para_FS_CC : Outport  Port=4
  sig_ST_msl : Outport  Port=5
  sig_CK_ParaLoad_msl : Outport  Port=6
  sig_fault_ES_msl : Outport  Port=7
  sig_sprt_msl : Outport  Port=8
  wires:
  Selector7/1 -> sig_sprt_msl/1
  Selector6/1 -> sig_fault_ES_msl/1
  Selector5/1 -> sig_CK_ParaLoad_msl/1
  Selector4/1 -> sig_ST_msl/1
  Selector3/1 -> Para_FS_CC/1
  Selector2/1 -> ins_FS_CC/1
  Selector1/1 -> ins_pwr_off_CC/1
  Selector/1 -> ins_pwr_on_CC/1
  Bus Selector1/4 -> Selector7/1  "<sig_sprt>"
  Bus Selector1/3 -> Selector6/1  "<sig_fault_ES>"
  Bus Selector1/2 -> Selector5/1  "<sig_CK_ParaLoad>"
  Bus Selector1/1 -> Selector4/1  "<sig_ST>"
  Bus Selector/4 -> Selector3/1  "<Para_FS>"
  Bus Selector/3 -> Selector2/1  "<ins_FS>"
  Bus Selector/2 -> Selector1/1  "<ins_pwr_of>"
  Bus Selector/1 -> Selector/1  "<ins_pwr_on>"
  sig_msl/1 -> Bus Selector1/1
  ins_CC/1 -> Bus Selector/1

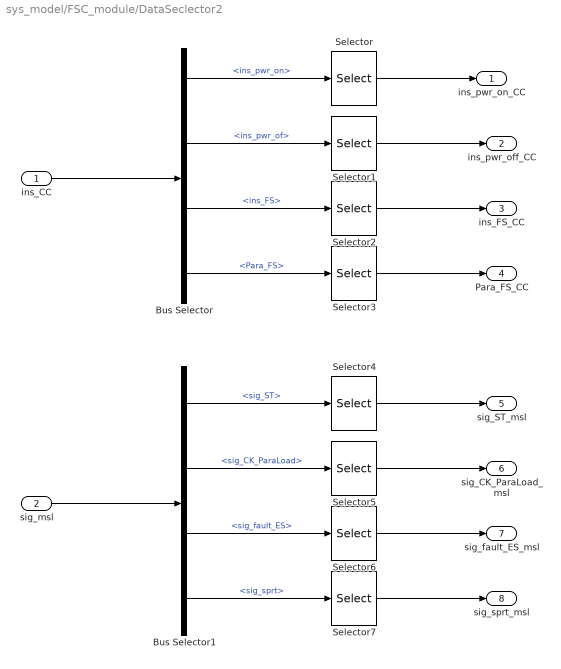
== system sys_model/FSC_module/DataSeclector2 ==
  ins_CC : Inport
  sig_msl : Inport  Port=2
  Bus Selector : BusSelector  OutputSignals=ins_pwr_on,ins_pwr_of,ins_FS,Para_FS
  Bus Selector1 : BusSelector  OutputSignals=sig_ST,sig_CK_ParaLoad,sig_fault_ES,sig_sprt
  Selector{,1..7} (8 alike) : Selector  InputPortWidth=8  Indices=[5 6]
  ins_pwr_on_CC : Outport
  ins_pwr_off_CC : Outport  Port=2
  ins_FS_CC : Outport  Port=3
  Para_FS_CC : Outport  Port=4
  sig_ST_msl : Outport  Port=5
  sig_CK_ParaLoad_msl : Outport  Port=6
  sig_fault_ES_msl : Outport  Port=7
  sig_sprt_msl : Outport  Port=8
  wires:
  ins_CC/1 -> Bus Selector/1
  sig_msl/1 -> Bus Selector1/1
  Bus Selector/1 -> Selector/1  "<ins_pwr_on>"
  Bus Selector/2 -> Selector1/1  "<ins_pwr_of>"
  Bus Selector/3 -> Selector2/1  "<ins_FS>"
  Bus Selector/4 -> Selector3/1  "<Para_FS>"
  Bus Selector1/1 -> Selector4/1  "<sig_ST>"
  Bus Selector1/2 -> Selector5/1  "<sig_CK_ParaLoad>"
  Bus Selector1/3 -> Selector6/1  "<sig_fault_ES>"
  Bus Selector1/4 -> Selector7/1  "<sig_sprt>"
  Selector/1 -> ins_pwr_on_CC/1
  Selector1/1 -> ins_pwr_off_CC/1
  Selector2/1 -> ins_FS_CC/1
  Selector3/1 -> Para_FS_CC/1
  Selector4/1 -> sig_ST_msl/1
  Selector5/1 -> sig_CK_ParaLoad_msl/1
  Selector6/1 -> sig_fault_ES_msl/1
  Selector7/1 -> sig_sprt_msl/1

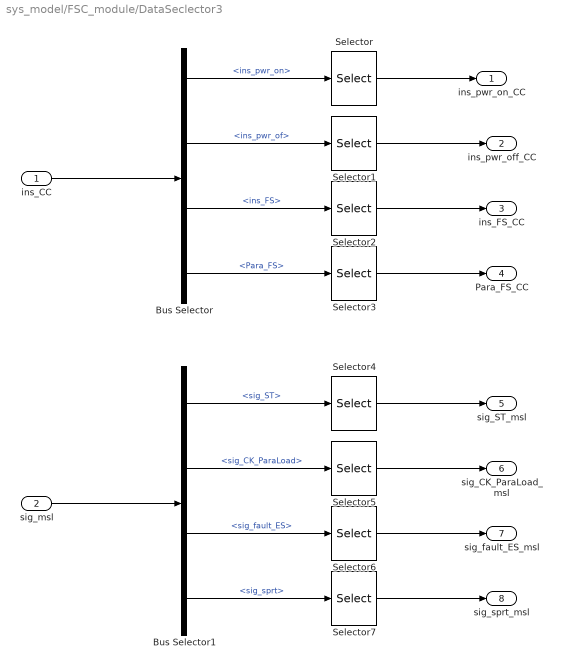
== system sys_model/FSC_module/DataSeclector3 ==
  ins_CC : Inport
  sig_msl : Inport  Port=2
  Bus Selector : BusSelector  OutputSignals=ins_pwr_on,ins_pwr_of,ins_FS,Para_FS
  Bus Selector1 : BusSelector  OutputSignals=sig_ST,sig_CK_ParaLoad,sig_fault_ES,sig_sprt
  Selector{,1..7} (8 alike) : Selector  InputPortWidth=8  Indices=[7 8]
  ins_pwr_on_CC : Outport
  ins_pwr_off_CC : Outport  Port=2
  ins_FS_CC : Outport  Port=3
  Para_FS_CC : Outport  Port=4
  sig_ST_msl : Outport  Port=5
  sig_CK_ParaLoad_msl : Outport  Port=6
  sig_fault_ES_msl : Outport  Port=7
  sig_sprt_msl : Outport  Port=8
  wires:
  Selector7/1 -> sig_sprt_msl/1
  Selector6/1 -> sig_fault_ES_msl/1
  Selector5/1 -> sig_CK_ParaLoad_msl/1
  Selector4/1 -> sig_ST_msl/1
  Selector3/1 -> Para_FS_CC/1
  Selector2/1 -> ins_FS_CC/1
  Selector1/1 -> ins_pwr_off_CC/1
  Selector/1 -> ins_pwr_on_CC/1
  Bus Selector1/4 -> Selector7/1  "<sig_sprt>"
  Bus Selector1/3 -> Selector6/1  "<sig_fault_ES>"
  Bus Selector1/2 -> Selector5/1  "<sig_CK_ParaLoad>"
  Bus Selector1/1 -> Selector4/1  "<sig_ST>"
  Bus Selector/4 -> Selector3/1  "<Para_FS>"
  Bus Selector/3 -> Selector2/1  "<ins_FS>"
  Bus Selector/2 -> Selector1/1  "<ins_pwr_of>"
  Bus Selector/1 -> Selector/1  "<ins_pwr_on>"
  sig_msl/1 -> Bus Selector1/1
  ins_CC/1 -> Bus Selector/1

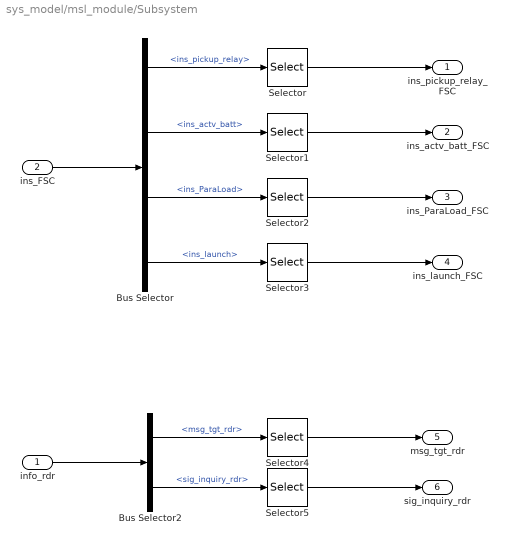
== system sys_model/msl_module/Subsystem ==
  info_rdr : Inport
  ins_FSC : Inport  Port=2
  Bus Selector : BusSelector  OutputSignals=ins_pickup_relay,ins_actv_batt,ins_ParaLoad,ins_launch
  Bus Selector2 : BusSelector  OutputSignals=msg_tgt_rdr,sig_inquiry_rdr
  Selector{,1..5} (6 alike) : Selector  InputPortWidth=8  Indices=[1]
  ins_pickup_relay_FSC : Outport
  ins_actv_batt_FSC : Outport  Port=2
  ins_ParaLoad_FSC : Outport  Port=3
  ins_launch_FSC : Outport  Port=4
  msg_tgt_rdr : Outport  Port=5
  sig_inquiry_rdr : Outport  Port=6
  wires:
  ins_FSC/1 -> Bus Selector/1
  Bus Selector/1 -> Selector/1  "<ins_pickup_relay>"
  Selector/1 -> ins_pickup_relay_FSC/1
  Bus Selector/2 -> Selector1/1  "<ins_actv_batt>"
  Selector1/1 -> ins_actv_batt_FSC/1
  Bus Selector/3 -> Selector2/1  "<ins_ParaLoad>"
  Bus Selector/4 -> Selector3/1  "<ins_launch>"
  Selector2/1 -> ins_ParaLoad_FSC/1
  Selector3/1 -> ins_launch_FSC/1
  info_rdr/1 -> Bus Selector2/1
  Bus Selector2/2 -> Selector5/1  "<sig_inquiry_rdr>"
  Bus Selector2/1 -> Selector4/1  "<msg_tgt_rdr>"
  Selector4/1 -> msg_tgt_rdr/1
  Selector5/1 -> sig_inquiry_rdr/1

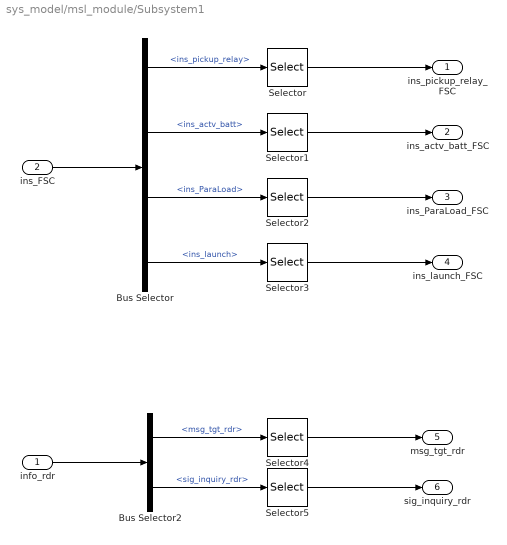
== system sys_model/msl_module/Subsystem1 ==
  info_rdr : Inport
  ins_FSC : Inport  Port=2
  Bus Selector : BusSelector  OutputSignals=ins_pickup_relay,ins_actv_batt,ins_ParaLoad,ins_launch
  Bus Selector2 : BusSelector  OutputSignals=msg_tgt_rdr,sig_inquiry_rdr
  Selector{,1..5} (6 alike) : Selector  InputPortWidth=8  Indices=2
  ins_pickup_relay_FSC : Outport
  ins_actv_batt_FSC : Outport  Port=2
  ins_ParaLoad_FSC : Outport  Port=3
  ins_launch_FSC : Outport  Port=4
  msg_tgt_rdr : Outport  Port=5
  sig_inquiry_rdr : Outport  Port=6
  wires:
  Selector5/1 -> sig_inquiry_rdr/1
  Selector4/1 -> msg_tgt_rdr/1
  Bus Selector2/1 -> Selector4/1  "<msg_tgt_rdr>"
  Bus Selector2/2 -> Selector5/1  "<sig_inquiry_rdr>"
  info_rdr/1 -> Bus Selector2/1
  Selector3/1 -> ins_launch_FSC/1
  Selector2/1 -> ins_ParaLoad_FSC/1
  Bus Selector/4 -> Selector3/1  "<ins_launch>"
  Bus Selector/3 -> Selector2/1  "<ins_ParaLoad>"
  Selector1/1 -> ins_actv_batt_FSC/1
  Bus Selector/2 -> Selector1/1  "<ins_actv_batt>"
  Selector/1 -> ins_pickup_relay_FSC/1
  Bus Selector/1 -> Selector/1  "<ins_pickup_relay>"
  ins_FSC/1 -> Bus Selector/1

== system sys_model/msl_module/Subsystem2 ==
  info_rdr : Inport
  ins_FSC : Inport  Port=2
  Bus Selector : BusSelector  OutputSignals=ins_pickup_relay,ins_actv_batt,ins_ParaLoad,ins_launch
  Bus Selector2 : BusSelector  OutputSignals=msg_tgt_rdr,sig_inquiry_rdr
  Selector{,1..5} (6 alike) : Selector  InputPortWidth=8  Indices=3
  ins_pickup_relay_FSC : Outport
  ins_actv_batt_FSC : Outport  Port=2
  ins_ParaLoad_FSC : Outport  Port=3
  ins_launch_FSC : Outport  Port=4
  msg_tgt_rdr : Outport  Port=5
  sig_inquiry_rdr : Outport  Port=6
  wires:
  ins_FSC/1 -> Bus Selector/1
  Bus Selector/1 -> Selector/1  "<ins_pickup_relay>"
  Selector/1 -> ins_pickup_relay_FSC/1
  Bus Selector/2 -> Selector1/1  "<ins_actv_batt>"
  Selector1/1 -> ins_actv_batt_FSC/1
  Bus Selector/3 -> Selector2/1  "<ins_ParaLoad>"
  Bus Selector/4 -> Selector3/1  "<ins_launch>"
  Selector2/1 -> ins_ParaLoad_FSC/1
  Selector3/1 -> ins_launch_FSC/1
  info_rdr/1 -> Bus Selector2/1
  Bus Selector2/2 -> Selector5/1  "<sig_inquiry_rdr>"
  Bus Selector2/1 -> Selector4/1  "<msg_tgt_rdr>"
  Selector4/1 -> msg_tgt_rdr/1
  Selector5/1 -> sig_inquiry_rdr/1

== system sys_model/msl_module/Subsystem3 ==
  info_rdr : Inport
  ins_FSC : Inport  Port=2
  Bus Selector : BusSelector  OutputSignals=ins_pickup_relay,ins_actv_batt,ins_ParaLoad,ins_launch
  Bus Selector2 : BusSelector  OutputSignals=msg_tgt_rdr,sig_inquiry_rdr
  Selector{,1..5} (6 alike) : Selector  InputPortWidth=8  Indices=4
  ins_pickup_relay_FSC : Outport
  ins_actv_batt_FSC : Outport  Port=2
  ins_ParaLoad_FSC : Outport  Port=3
  ins_launch_FSC : Outport  Port=4
  msg_tgt_rdr : Outport  Port=5
  sig_inquiry_rdr : Outport  Port=6
  wires:
  Selector5/1 -> sig_inquiry_rdr/1
  Selector4/1 -> msg_tgt_rdr/1
  Bus Selector2/1 -> Selector4/1  "<msg_tgt_rdr>"
  Bus Selector2/2 -> Selector5/1  "<sig_inquiry_rdr>"
  info_rdr/1 -> Bus Selector2/1
  Selector3/1 -> ins_launch_FSC/1
  Selector2/1 -> ins_ParaLoad_FSC/1
  Bus Selector/4 -> Selector3/1  "<ins_launch>"
  Bus Selector/3 -> Selector2/1  "<ins_ParaLoad>"
  Selector1/1 -> ins_actv_batt_FSC/1
  Bus Selector/2 -> Selector1/1  "<ins_actv_batt>"
  Selector/1 -> ins_pickup_relay_FSC/1
  Bus Selector/1 -> Selector/1  "<ins_pickup_relay>"
  ins_FSC/1 -> Bus Selector/1

== system sys_model/msl_module/Subsystem4 ==
  info_rdr : Inport
  ins_FSC : Inport  Port=2
  Bus Selector : BusSelector  OutputSignals=ins_pickup_relay,ins_actv_batt,ins_ParaLoad,ins_launch
  Bus Selector2 : BusSelector  OutputSignals=msg_tgt_rdr,sig_inquiry_rdr
  Selector{,1..5} (6 alike) : Selector  InputPortWidth=8  Indices=5
  ins_pickup_relay_FSC : Outport
  ins_actv_batt_FSC : Outport  Port=2
  ins_ParaLoad_FSC : Outport  Port=3
  ins_launch_FSC : Outport  Port=4
  msg_tgt_rdr : Outport  Port=5
  sig_inquiry_rdr : Outport  Port=6
  wires:
  ins_FSC/1 -> Bus Selector/1
  Bus Selector/1 -> Selector/1  "<ins_pickup_relay>"
  Selector/1 -> ins_pickup_relay_FSC/1
  Bus Selector/2 -> Selector1/1  "<ins_actv_batt>"
  Selector1/1 -> ins_actv_batt_FSC/1
  Bus Selector/3 -> Selector2/1  "<ins_ParaLoad>"
  Bus Selector/4 -> Selector3/1  "<ins_launch>"
  Selector2/1 -> ins_ParaLoad_FSC/1
  Selector3/1 -> ins_launch_FSC/1
  info_rdr/1 -> Bus Selector2/1
  Bus Selector2/2 -> Selector5/1  "<sig_inquiry_rdr>"
  Bus Selector2/1 -> Selector4/1  "<msg_tgt_rdr>"
  Selector4/1 -> msg_tgt_rdr/1
  Selector5/1 -> sig_inquiry_rdr/1

== system sys_model/msl_module/Subsystem5 ==
  info_rdr : Inport
  ins_FSC : Inport  Port=2
  Bus Selector : BusSelector  OutputSignals=ins_pickup_relay,ins_actv_batt,ins_ParaLoad,ins_launch
  Bus Selector2 : BusSelector  OutputSignals=msg_tgt_rdr,sig_inquiry_rdr
  Selector{,1..5} (6 alike) : Selector  InputPortWidth=8  Indices=6
  ins_pickup_relay_FSC : Outport
  ins_actv_batt_FSC : Outport  Port=2
  ins_ParaLoad_FSC : Outport  Port=3
  ins_launch_FSC : Outport  Port=4
  msg_tgt_rdr : Outport  Port=5
  sig_inquiry_rdr : Outport  Port=6
  wires:
  Selector5/1 -> sig_inquiry_rdr/1
  Selector4/1 -> msg_tgt_rdr/1
  Bus Selector2/1 -> Selector4/1  "<msg_tgt_rdr>"
  Bus Selector2/2 -> Selector5/1  "<sig_inquiry_rdr>"
  info_rdr/1 -> Bus Selector2/1
  Selector3/1 -> ins_launch_FSC/1
  Selector2/1 -> ins_ParaLoad_FSC/1
  Bus Selector/4 -> Selector3/1  "<ins_launch>"
  Bus Selector/3 -> Selector2/1  "<ins_ParaLoad>"
  Selector1/1 -> ins_actv_batt_FSC/1
  Bus Selector/2 -> Selector1/1  "<ins_actv_batt>"
  Selector/1 -> ins_pickup_relay_FSC/1
  Bus Selector/1 -> Selector/1  "<ins_pickup_relay>"
  ins_FSC/1 -> Bus Selector/1

== system sys_model/msl_module/Subsystem6 ==
  info_rdr : Inport
  ins_FSC : Inport  Port=2
  Bus Selector : BusSelector  OutputSignals=ins_pickup_relay,ins_actv_batt,ins_ParaLoad,ins_launch
  Bus Selector2 : BusSelector  OutputSignals=msg_tgt_rdr,sig_inquiry_rdr
  Selector : Selector  InputPortWidth=8  Indices=7
  Selector{1..5} (5 alike) : Selector  InputPortWidth=8  Indices=6
  ins_pickup_relay_FSC : Outport
  ins_actv_batt_FSC : Outport  Port=2
  ins_ParaLoad_FSC : Outport  Port=3
  ins_launch_FSC : Outport  Port=4
  msg_tgt_rdr : Outport  Port=5
  sig_inquiry_rdr : Outport  Port=6
  wires:
  ins_FSC/1 -> Bus Selector/1
  Bus Selector/1 -> Selector/1  "<ins_pickup_relay>"
  Selector/1 -> ins_pickup_relay_FSC/1
  Bus Selector/2 -> Selector1/1  "<ins_actv_batt>"
  Selector1/1 -> ins_actv_batt_FSC/1
  Bus Selector/3 -> Selector2/1  "<ins_ParaLoad>"
  Bus Selector/4 -> Selector3/1  "<ins_launch>"
  Selector2/1 -> ins_ParaLoad_FSC/1
  Selector3/1 -> ins_launch_FSC/1
  info_rdr/1 -> Bus Selector2/1
  Bus Selector2/2 -> Selector5/1  "<sig_inquiry_rdr>"
  Bus Selector2/1 -> Selector4/1  "<msg_tgt_rdr>"
  Selector4/1 -> msg_tgt_rdr/1
  Selector5/1 -> sig_inquiry_rdr/1

== system sys_model/msl_module/Subsystem7 ==
  info_rdr : Inport
  ins_FSC : Inport  Port=2
  Bus Selector : BusSelector  OutputSignals=ins_pickup_relay,ins_actv_batt,ins_ParaLoad,ins_launch
  Bus Selector2 : BusSelector  OutputSignals=msg_tgt_rdr,sig_inquiry_rdr
  Selector{1..6} (6 alike) : Selector  InputPortWidth=8  Indices=8
  ins_pickup_relay_FSC : Outport  OutDataTypeStr=boolean
  ins_actv_batt_FSC : Outport  Port=2  OutDataTypeStr=boolean
  ins_ParaLoad_FSC : Outport  Port=3  OutDataTypeStr=boolean
  ins_launch_FSC : Outport  Port=4
  msg_tgt_rdr : Outport  Port=5
  sig_inquiry_rdr : Outport  Port=6
  wires:
  Selector5/1 -> sig_inquiry_rdr/1
  Selector4/1 -> msg_tgt_rdr/1
  Bus Selector2/1 -> Selector4/1  "<msg_tgt_rdr>"
  Bus Selector2/2 -> Selector5/1  "<sig_inquiry_rdr>"
  info_rdr/1 -> Bus Selector2/1
  Selector3/1 -> ins_launch_FSC/1
  Selector2/1 -> ins_ParaLoad_FSC/1
  Bus Selector/4 -> Selector3/1  "<ins_launch>"
  Bus Selector/3 -> Selector2/1  "<ins_ParaLoad>"
  Selector1/1 -> ins_actv_batt_FSC/1
  Bus Selector/2 -> Selector1/1  "<ins_actv_batt>"
  Selector6/1 -> ins_pickup_relay_FSC/1
  Bus Selector/1 -> Selector6/1  "<ins_pickup_relay>"
  ins_FSC/1 -> Bus Selector/1

== system sys_model/CC_module/Subsystem/Subsystem ==
  ins_fs : Inport
  LDData : Inport  Port=2
  AsnData : Inport  Port=3
  Bus Selector : BusSelector  OutputSignals=Pos
  Bus Selector1 : BusSelector  OutputSignals=Pos
  Chart : Stateflow chart  TreatAsAtomicUnit=on
  Chart1 : Stateflow chart  TreatAsAtomicUnit=on
  Display : Display
  Display1 : Display
  Terminator : Terminator
  mslMotion : Subsystem  TreatAsAtomicUnit=on
  MslMotion : Outport  OutDataTypeStr=Bus: MslDataBusObject
  wires:
  AsnData/1 -> Chart/1(AsnData)
  Chart/1(MsltgtInd) -> Terminator/1
  Chart/2(FSMsltgtInd) -> mslMotion/1(FSMsltgtInd), Chart1/1(FSMsltgtInd)
  ins_fs/1 -> Chart/2(ins_fs)
  LDData/1 -> mslMotion/2(LDData)
  Chart1/1(MslMotion) -> Bus Selector/1, MslMotion/1
  Bus Selector/1 -> Display/1  "<Pos>"
  mslMotion/1(MslMotionNew) -> Bus Selector1/1, Chart1/2(MslMotionNew)
  Bus Selector1/1 -> Display1/1  "<Pos>"

== system sys_model/CC_module/input/For Each Subsystem ==
  In1 : Inport  Partition=on  PartitionDimension=1  PartitionWidth=1
  Bus Selector : BusSelector  OutputSignals=pos,vel
  For Each : ForEach  DisableCoverage=on  IndexMode=One-based
  pos : Outport  ConcatenationDimension=2
  vel : Outport  Port=2  ConcatenationDimension=2
  wires:
  Bus Selector/2 -> vel/1  "<vel>"
  In1/1 -> Bus Selector/1
  Bus Selector/1 -> pos/1  "<pos>"

== system sys_model/CC_module/input/TargetGeneration ==
  Constant3 : Constant  Value=Vtgt*200
  Integrator : Integrator
  Pos : Outport
  Vel : Outport  Port=2
  wires:
  Constant3/1 -> Vel/1, Integrator/1  "Vel"
  Integrator/1 -> Pos/1  "Pos"

== system sys_model/CC_module/Subsystem/Subsystem/mslMotion ==
  FSMsltgtInd : Inport
  LDData : Inport  Port=2
  Bus Creator1 : BusCreator  Inputs=2  OutDataTypeStr=Bus: MslDataBusObject  NonVirtualBus=on
  Constant3 : Constant  Value=Vmsl*100  OutDataTypeStr=double
  Integrator : Integrator  InitialCondition=250*ones(8,2)
  Terminator : Terminator
  Terminator1 : Terminator
  MslMotionNew : Outport
  wires:
  FSMsltgtInd/1 -> Terminator1/1
  Constant3/1 -> Bus Creator1/2, Integrator/1  "Vel"
  LDData/1 -> Terminator/1
  Integrator/1 -> Bus Creator1/1  "Pos"
  Bus Creator1/1 -> MslMotionNew/1
